simulink model "model"  (R2016a)
(part 2 of 2)

  bus74 : powerlib/Measurements/Load Flow Bus  LConnTagsString=a  Phases=single  Connectors=on one side  ID=bus74  Vbase=225000  Vref=1  Vangle=0  VLF=1  VLFb=1  VLFc=1  angleLF=0  angleLFb=0  angleLFc=0
      settings: AttributesFormatString=|
      | %<ID>
      | %<Vbase>V
      | %<VLF>pu
      | %<angleLF>deg.
      | %<Name>
  bus75 : powerlib/Measurements/Load Flow Bus  LConnTagsString=a  Phases=single  Connectors=on one side  ID=bus75  Vbase=225000  Vref=1  Vangle=0  VLF=1  VLFb=1  VLFc=1  angleLF=0  angleLFb=0  angleLFc=0
      settings: AttributesFormatString=|
      | %<ID>
      | %<Vbase>V
      | %<VLF>pu
      | %<angleLF>deg.
      | %<Name>
  bus76 : powerlib/Measurements/Load Flow Bus  LConnTagsString=a  Phases=single  Connectors=on one side  ID=bus76  Vbase=225000  Vref=1  Vangle=0  VLF=1  VLFb=1  VLFc=1  angleLF=0  angleLFb=0  angleLFc=0
      settings: AttributesFormatString=|
      | %<ID>
      | %<Vbase>V
      | %<VLF>pu
      | %<angleLF>deg.
      | %<Name>
  bus77 : powerlib/Measurements/Load Flow Bus  LConnTagsString=a  Phases=single  Connectors=on one side  ID=bus77  Vbase=225000  Vref=1  Vangle=0  VLF=1  VLFb=1  VLFc=1  angleLF=0  angleLFb=0  angleLFc=0
      settings: AttributesFormatString=|
      | %<ID>
      | %<Vbase>V
      | %<VLF>pu
      | %<angleLF>deg.
      | %<Name>
  bus78 : powerlib/Measurements/Load Flow Bus  LConnTagsString=a  Phases=single  Connectors=on one side  ID=bus78  Vbase=225000  Vref=1  Vangle=0  VLF=1  VLFb=1  VLFc=1  angleLF=0  angleLFb=0  angleLFc=0
      settings: AttributesFormatString=|
      | %<ID>
      | %<Vbase>V
      | %<VLF>pu
      | %<angleLF>deg.
      | %<Name>
  bus79 : powerlib/Measurements/Load Flow Bus  LConnTagsString=a  Phases=single  Connectors=on one side  ID=bus79  Vbase=225000  Vref=1  Vangle=0  VLF=1  VLFb=1  VLFc=1  angleLF=0  angleLFb=0  angleLFc=0
      settings: AttributesFormatString=|
      | %<ID>
      | %<Vbase>V
      | %<VLF>pu
      | %<angleLF>deg.
      | %<Name>
  bus8 : powerlib/Measurements/Load Flow Bus  LConnTagsString=a  Phases=single  Connectors=on one side  ID=bus8  Vbase=225000  Vref=1  Vangle=0  VLF=1  VLFb=1  VLFc=1  angleLF=0  angleLFb=0  angleLFc=0
      settings: AttributesFormatString=|
      | %<ID>
      | %<Vbase>V
      | %<VLF>pu
      | %<angleLF>deg.
      | %<Name>
  bus80 : powerlib/Measurements/Load Flow Bus  LConnTagsString=a  Phases=single  Connectors=on one side  ID=bus80  Vbase=225000  Vref=1  Vangle=0  VLF=1  VLFb=1  VLFc=1  angleLF=0  angleLFb=0  angleLFc=0
      settings: AttributesFormatString=|
      | %<ID>
      | %<Vbase>V
      | %<VLF>pu
      | %<angleLF>deg.
      | %<Name>
  bus81 : powerlib/Measurements/Load Flow Bus  LConnTagsString=a  Phases=single  Connectors=on one side  ID=bus81  Vbase=225000  Vref=1  Vangle=0  VLF=1  VLFb=1  VLFc=1  angleLF=0  angleLFb=0  angleLFc=0
      settings: AttributesFormatString=|
      | %<ID>
      | %<Vbase>V
      | %<VLF>pu
      | %<angleLF>deg.
      | %<Name>
  bus82 : powerlib/Measurements/Load Flow Bus  LConnTagsString=a  Phases=single  Connectors=on one side  ID=bus82  Vbase=225000  Vref=1  Vangle=0  VLF=1  VLFb=1  VLFc=1  angleLF=0  angleLFb=0  angleLFc=0
      settings: AttributesFormatString=|
      | %<ID>
      | %<Vbase>V
      | %<VLF>pu
      | %<angleLF>deg.
      | %<Name>
  bus83 : powerlib/Measurements/Load Flow Bus  LConnTagsString=a  Phases=single  Connectors=on one side  ID=bus83  Vbase=225000  Vref=1  Vangle=0  VLF=1  VLFb=1  VLFc=1  angleLF=0  angleLFb=0  angleLFc=0
      settings: AttributesFormatString=|
      | %<ID>
      | %<Vbase>V
      | %<VLF>pu
      | %<angleLF>deg.
      | %<Name>
  bus84 : powerlib/Measurements/Load Flow Bus  LConnTagsString=a  Phases=single  Connectors=on one side  ID=bus84  Vbase=225000  Vref=1  Vangle=0  VLF=1  VLFb=1  VLFc=1  angleLF=0  angleLFb=0  angleLFc=0
      settings: AttributesFormatString=|
      | %<ID>
      | %<Vbase>V
      | %<VLF>pu
      | %<angleLF>deg.
      | %<Name>
  bus85 : powerlib/Measurements/Load Flow Bus  LConnTagsString=a  Phases=single  Connectors=on one side  ID=bus85  Vbase=225000  Vref=1  Vangle=0  VLF=1  VLFb=1  VLFc=1  angleLF=0  angleLFb=0  angleLFc=0
      settings: AttributesFormatString=|
      | %<ID>
      | %<Vbase>V
      | %<VLF>pu
      | %<angleLF>deg.
      | %<Name>
  bus86 : powerlib/Measurements/Load Flow Bus  LConnTagsString=a  Phases=single  Connectors=on one side  ID=bus86  Vbase=225000  Vref=1  Vangle=0  VLF=1  VLFb=1  VLFc=1  angleLF=0  angleLFb=0  angleLFc=0
      settings: AttributesFormatString=|
      | %<ID>
      | %<Vbase>V
      | %<VLF>pu
      | %<angleLF>deg.
      | %<Name>
  bus87 : powerlib/Measurements/Load Flow Bus  LConnTagsString=a  Phases=single  Connectors=on one side  ID=bus87  Vbase=225000  Vref=1  Vangle=0  VLF=1  VLFb=1  VLFc=1  angleLF=0  angleLFb=0  angleLFc=0
      settings: AttributesFormatString=|
      | %<ID>
      | %<Vbase>V
      | %<VLF>pu
      | %<angleLF>deg.
      | %<Name>
  bus88 : powerlib/Measurements/Load Flow Bus  LConnTagsString=a  Phases=single  Connectors=on one side  ID=bus88  Vbase=225000  Vref=1  Vangle=0  VLF=1  VLFb=1  VLFc=1  angleLF=0  angleLFb=0  angleLFc=0
      settings: AttributesFormatString=|
      | %<ID>
      | %<Vbase>V
      | %<VLF>pu
      | %<angleLF>deg.
      | %<Name>
  bus89 : powerlib/Measurements/Load Flow Bus  LConnTagsString=a  Phases=single  Connectors=on one side  ID=bus89  Vbase=225000  Vref=1  Vangle=0  VLF=1  VLFb=1  VLFc=1  angleLF=0  angleLFb=0  angleLFc=0
      settings: AttributesFormatString=|
      | %<ID>
      | %<Vbase>V
      | %<VLF>pu
      | %<angleLF>deg.
      | %<Name>
  bus9 : powerlib/Measurements/Load Flow Bus  LConnTagsString=a  Phases=single  Connectors=on one side  ID=bus9  Vbase=225000  Vref=1  Vangle=0  VLF=1  VLFb=1  VLFc=1  angleLF=0  angleLFb=0  angleLFc=0
      settings: AttributesFormatString=|
      | %<ID>
      | %<Vbase>V
      | %<VLF>pu
      | %<angleLF>deg.
      | %<Name>
  bus90 : powerlib/Measurements/Load Flow Bus  LConnTagsString=a  Phases=single  Connectors=on one side  ID=bus90  Vbase=225000  Vref=1  Vangle=0  VLF=1  VLFb=1  VLFc=1  angleLF=0  angleLFb=0  angleLFc=0
      settings: AttributesFormatString=|
      | %<ID>
      | %<Vbase>V
      | %<VLF>pu
      | %<angleLF>deg.
      | %<Name>
  bus91 : powerlib/Measurements/Load Flow Bus  LConnTagsString=a  Phases=single  Connectors=on one side  ID=bus91  Vbase=225000  Vref=1  Vangle=0  VLF=1  VLFb=1  VLFc=1  angleLF=0  angleLFb=0  angleLFc=0
      settings: AttributesFormatString=|
      | %<ID>
      | %<Vbase>V
      | %<VLF>pu
      | %<angleLF>deg.
      | %<Name>
  bus92 : powerlib/Measurements/Load Flow Bus  LConnTagsString=a  Phases=single  Connectors=on one side  ID=bus92  Vbase=225000  Vref=1  Vangle=0  VLF=1  VLFb=1  VLFc=1  angleLF=0  angleLFb=0  angleLFc=0
      settings: AttributesFormatString=|
      | %<ID>
      | %<Vbase>V
      | %<VLF>pu
      | %<angleLF>deg.
      | %<Name>
  bus93 : powerlib/Measurements/Load Flow Bus  LConnTagsString=a  Phases=single  Connectors=on one side  ID=bus93  Vbase=225000  Vref=1  Vangle=0  VLF=1  VLFb=1  VLFc=1  angleLF=0  angleLFb=0  angleLFc=0
      settings: AttributesFormatString=|
      | %<ID>
      | %<Vbase>V
      | %<VLF>pu
      | %<angleLF>deg.
      | %<Name>
  bus94 : powerlib/Measurements/Load Flow Bus  LConnTagsString=a  Phases=single  Connectors=on one side  ID=bus94  Vbase=225000  Vref=1  Vangle=0  VLF=1  VLFb=1  VLFc=1  angleLF=0  angleLFb=0  angleLFc=0
      settings: AttributesFormatString=|
      | %<ID>
      | %<Vbase>V
      | %<VLF>pu
      | %<angleLF>deg.
      | %<Name>
  bus95 : powerlib/Measurements/Load Flow Bus  LConnTagsString=a  Phases=single  Connectors=on one side  ID=bus95  Vbase=225000  Vref=1  Vangle=0  VLF=1  VLFb=1  VLFc=1  angleLF=0  angleLFb=0  angleLFc=0
      settings: AttributesFormatString=|
      | %<ID>
      | %<Vbase>V
      | %<VLF>pu
      | %<angleLF>deg.
      | %<Name>
  bus96 : powerlib/Measurements/Load Flow Bus  LConnTagsString=a  Phases=single  Connectors=on one side  ID=bus96  Vbase=225000  Vref=1  Vangle=0  VLF=1  VLFb=1  VLFc=1  angleLF=0  angleLFb=0  angleLFc=0
      settings: AttributesFormatString=|
      | %<ID>
      | %<Vbase>V
      | %<VLF>pu
      | %<angleLF>deg.
      | %<Name>
  bus97 : powerlib/Measurements/Load Flow Bus  LConnTagsString=a  Phases=single  Connectors=on one side  ID=bus97  Vbase=225000  Vref=1  Vangle=0  VLF=1  VLFb=1  VLFc=1  angleLF=0  angleLFb=0  angleLFc=0
      settings: AttributesFormatString=|
      | %<ID>
      | %<Vbase>V
      | %<VLF>pu
      | %<angleLF>deg.
      | %<Name>
  bus98 : powerlib/Measurements/Load Flow Bus  LConnTagsString=a  Phases=single  Connectors=on one side  ID=bus98  Vbase=225000  Vref=1  Vangle=0  VLF=1  VLFb=1  VLFc=1  angleLF=0  angleLFb=0  angleLFc=0
      settings: AttributesFormatString=|
      | %<ID>
      | %<Vbase>V
      | %<VLF>pu
      | %<angleLF>deg.
      | %<Name>
  bus99 : powerlib/Measurements/Load Flow Bus  LConnTagsString=a  Phases=single  Connectors=on one side  ID=bus99  Vbase=225000  Vref=1  Vangle=0  VLF=1  VLFb=1  VLFc=1  angleLF=0  angleLFb=0  angleLFc=0
      settings: AttributesFormatString=|
      | %<ID>
      | %<Vbase>V
      | %<VLF>pu
      | %<angleLF>deg.
      | %<Name>
  powergui : powerlib/powergui  Priority=1  SimulationMode=Phasor  SolverType=Tustin/Backward Euler (TBE)  SampleTime=50e-6  frequency=50  SPID=off  DisableSnubberDevices=off  DisableRonSwitches=off  DisableVfSwitches=off  SwTol=0  DisplayEquations=off  Interpol=off  ExternalGateDelay=off  methode=off  Ts=10  FunctionMessages=off  echomessages=off  HookPort=off  EnableUseOfTLC=off  x0status=blocks  frequencyindice=50  Pbase=3000e6  ErrMax=0.0001  Iterations=50  UnitsV=V  UnitsW=W  buscounter=0  RestoreLinks=warning  ResistiveCurrentMeasurement=off  Frange=[0:2:500]  Ylog=off  Xlog=on  ShowGrid=off  save=off  variable=ZData  structure=0  ZoomFFT=off  StartTime=0.0  cycles=1  DisplayStyle=1  fundamental=60  FreqAxis=off  MaxFrequency=1000  frequencyindicesteady=1  RmsSteady=1  display=off
  connections:
  _CN_200906153_225000_CN_250878457_225000/LConn1 -- T_200906153_225000_/LConn1 -- _CN_200906153_225000_CN_285708473_225000/LConn1 -- _CN_200906153_225000_CN_218739270_225000/LConn1 -- _CN_200906153_225000_CN_271316486_225000/LConn1
  _CN_200906153_225000_CN_250878457_225000/LConn2 -- T_200906153_225000_/LConn2 -- _CN_200906153_225000_CN_285708473_225000/LConn2 -- _CN_200906153_225000_CN_218739270_225000/LConn2 -- _CN_200906153_225000_CN_271316486_225000/LConn2
  _CN_200906153_225000_CN_250878457_225000/LConn3 -- T_200906153_225000_/LConn3 -- _CN_200906153_225000_CN_285708473_225000/LConn3 -- _CN_200906153_225000_CN_218739270_225000/LConn3 -- _CN_200906153_225000_CN_271316486_225000/LConn3 -- bus1/LConn1
  _CN_200906153_225000_CN_250878457_225000/RConn1 -- T_250878457_225000_/LConn1 -- _CN_94548360_225000_CN_250878457_225000/LConn1 -- _CN_208002693_225000_CN_250878457_225000/LConn1
  _CN_200906153_225000_CN_250878457_225000/RConn2 -- T_250878457_225000_/LConn2 -- _CN_94548360_225000_CN_250878457_225000/LConn2 -- _CN_208002693_225000_CN_250878457_225000/LConn2
  _CN_200906153_225000_CN_250878457_225000/RConn3 -- T_250878457_225000_/LConn3 -- _CN_94548360_225000_CN_250878457_225000/LConn3 -- bus2/LConn1 -- _CN_208002693_225000_CN_250878457_225000/LConn3
  T_285708473_225000_/LConn1 -- _CN_200906153_225000_CN_285708473_225000/RConn1
  T_285708473_225000_/LConn2 -- _CN_200906153_225000_CN_285708473_225000/RConn2
  _CN_200906153_225000_CN_285708473_225000/RConn3 -- T_285708473_225000_/LConn3 -- bus3/LConn1
  T_218739270_225000_/LConn1 -- _CN_200906153_225000_CN_218739270_225000/RConn1
  T_218739270_225000_/LConn2 -- _CN_200906153_225000_CN_218739270_225000/RConn2
  _CN_200906153_225000_CN_218739270_225000/RConn3 -- T_218739270_225000_/LConn3 -- bus4/LConn1
  T_271316486_225000_/LConn1 -- _CN_200906153_225000_CN_271316486_225000/RConn1
  T_271316486_225000_/LConn2 -- _CN_200906153_225000_CN_271316486_225000/RConn2
  _CN_200906153_225000_CN_271316486_225000/RConn3 -- T_271316486_225000_/LConn3 -- bus5/LConn1
  _CN_97706499_225000_CN_215403934_225000/LConn1 -- T_97706499_225000_/RConn1 -- _CN_97706499_225000_CN_94548360_225000/LConn1 -- L_97706499/LConn1 -- _CN_97706499_225000_CN_320483882_225000/LConn1 -- _CN_97706499_225000_CN_316738277_225000/LConn1 -- _CN_97706499_225000_CN_200913450_225000/LConn1 -- _CN_97706499_225000_CN_182345278_225000/LConn1
  _CN_97706499_225000_CN_215403934_225000/LConn2 -- T_97706499_225000_/RConn2 -- _CN_97706499_225000_CN_94548360_225000/LConn2 -- L_97706499/LConn2 -- _CN_97706499_225000_CN_320483882_225000/LConn2 -- _CN_97706499_225000_CN_316738277_225000/LConn2 -- _CN_97706499_225000_CN_200913450_225000/LConn2 -- _CN_97706499_225000_CN_182345278_225000/LConn2
  _CN_97706499_225000_CN_215403934_225000/LConn3 -- T_97706499_225000_/RConn3 -- _CN_97706499_225000_CN_94548360_225000/LConn3 -- L_97706499/LConn3 -- bus6/LConn1 -- _CN_97706499_225000_CN_320483882_225000/LConn3 -- _CN_97706499_225000_CN_316738277_225000/LConn3 -- _CN_97706499_225000_CN_200913450_225000/LConn3 -- _CN_97706499_225000_CN_182345278_225000/LConn3
  _CN_97706499_225000_CN_215403934_225000/RConn1 -- T_215403934_225000_/LConn1 -- _CN_94548360_225000_CN_215403934_225000/LConn1
  _CN_97706499_225000_CN_215403934_225000/RConn2 -- T_215403934_225000_/LConn2 -- _CN_94548360_225000_CN_215403934_225000/LConn2
  _CN_97706499_225000_CN_215403934_225000/RConn3 -- T_215403934_225000_/LConn3 -- _CN_94548360_225000_CN_215403934_225000/LConn3 -- bus7/LConn1
  T_320483882_225000_/LConn1 -- _CN_97706499_225000_CN_320483882_225000/RConn1
  T_320483882_225000_/LConn2 -- _CN_97706499_225000_CN_320483882_225000/RConn2
  _CN_97706499_225000_CN_320483882_225000/RConn3 -- T_320483882_225000_/LConn3 -- bus8/LConn1
  _CN_97706499_225000_CN_316738277_225000/RConn1 -- T_316738277__/RConn1 -- L_316738277/LConn1
  _CN_97706499_225000_CN_316738277_225000/RConn2 -- T_316738277__/RConn2 -- L_316738277/LConn2
  _CN_97706499_225000_CN_316738277_225000/RConn3 -- T_316738277__/RConn3 -- L_316738277/LConn3 -- bus9/LConn1
  _CN_97706499_225000_CN_200913450_225000/RConn1 -- T_200913450_225000_/LConn1 -- _CN_200913450_225000_CN_200915133_225000/LConn1 -- _CN_200913450_225000_CN_197830862_225000/LConn1
  _CN_97706499_225000_CN_200913450_225000/RConn2 -- T_200913450_225000_/LConn2 -- _CN_200913450_225000_CN_200915133_225000/LConn2 -- _CN_200913450_225000_CN_197830862_225000/LConn2
  _CN_97706499_225000_CN_200913450_225000/RConn3 -- T_200913450_225000_/LConn3 -- _CN_200913450_225000_CN_200915133_225000/LConn3 -- _CN_200913450_225000_CN_197830862_225000/LConn3 -- bus10/LConn1
  _CN_97706499_225000_CN_182345278_225000/RConn1 -- T_182345278_225000_/LConn1 -- _CN_200915133_225000_CN_182345278_225000/LConn1
  _CN_97706499_225000_CN_182345278_225000/RConn2 -- T_182345278_225000_/LConn2 -- _CN_200915133_225000_CN_182345278_225000/LConn2
  _CN_97706499_225000_CN_182345278_225000/RConn3 -- T_182345278_225000_/LConn3 -- _CN_200915133_225000_CN_182345278_225000/LConn3 -- bus11/LConn1
  _CN_97706499_225000_CN_94548360_225000/RConn1 -- T_94548360_225000_/LConn1 -- _CN_94548360_225000_CN_215403934_225000/RConn1 -- _CN_94548360_225000_CN_250878457_225000/RConn1
  _CN_97706499_225000_CN_94548360_225000/RConn2 -- T_94548360_225000_/LConn2 -- _CN_94548360_225000_CN_215403934_225000/RConn2 -- _CN_94548360_225000_CN_250878457_225000/RConn2
  _CN_97706499_225000_CN_94548360_225000/RConn3 -- T_94548360_225000_/LConn3 -- _CN_94548360_225000_CN_215403934_225000/RConn3 -- bus12/LConn1 -- _CN_94548360_225000_CN_250878457_225000/RConn3
  _CN_208002693_225000_CN_108482559_225000/LConn1 -- T_208002693_225000_/LConn1 -- _CN_208002693_225000_CN_250878457_225000/RConn1 -- _CN_208002693_225000_CN_131995387_225000/LConn1
  _CN_208002693_225000_CN_108482559_225000/LConn2 -- T_208002693_225000_/LConn2 -- _CN_208002693_225000_CN_250878457_225000/RConn2 -- _CN_208002693_225000_CN_131995387_225000/LConn2
  _CN_208002693_225000_CN_108482559_225000/LConn3 -- T_208002693_225000_/LConn3 -- _CN_208002693_225000_CN_250878457_225000/RConn3 -- _CN_208002693_225000_CN_131995387_225000/LConn3 -- bus13/LConn1
  T_108482559_225000_/LConn1 -- _CN_208002693_225000_CN_108482559_225000/RConn1
  T_108482559_225000_/LConn2 -- _CN_208002693_225000_CN_108482559_225000/RConn2
  _CN_208002693_225000_CN_108482559_225000/RConn3 -- T_108482559_225000_/LConn3 -- bus14/LConn1
  _CN_208002693_225000_CN_131995387_225000/RConn1 -- T_131995387_225000_/LConn1 -- _CN_131992905_225000_CN_131995387_225000/LConn1 -- _CN_131995387_225000_CN_131408509_225000/LConn1
  _CN_208002693_225000_CN_131995387_225000/RConn2 -- T_131995387_225000_/LConn2 -- _CN_131992905_225000_CN_131995387_225000/LConn2 -- _CN_131995387_225000_CN_131408509_225000/LConn2
  _CN_208002693_225000_CN_131995387_225000/RConn3 -- T_131995387_225000_/LConn3 -- _CN_131992905_225000_CN_131995387_225000/LConn3 -- _CN_131995387_225000_CN_131408509_225000/LConn3 -- bus15/LConn1
  _CN_131891079_225000_CN_131892127_225000/LConn1 -- T_131891079_225000;60000_/LConn1 -- _CN_131891079_225000_CN_95436126_225000/LConn1 -- _CN_131891079_225000_CN_207991977_225000/LConn1 -- _CN_131891079_225000_CN_131946012_225000/LConn1 -- _CN_131891079_225000_CN_131408509_225000/LConn1 -- _CN_131891079_225000_CN_131588990_225000/LConn1 -- _CN_131891079_225000_CN_131267165_225000/LConn1 -- _CN_131891079_225000_CN_143628748_225000/LConn1 -- _CN_131891079_225000_CN_131902940_225000/LConn1
  _CN_131891079_225000_CN_131892127_225000/LConn2 -- T_131891079_225000;60000_/LConn2 -- _CN_131891079_225000_CN_95436126_225000/LConn2 -- _CN_131891079_225000_CN_207991977_225000/LConn2 -- _CN_131891079_225000_CN_131946012_225000/LConn2 -- _CN_131891079_225000_CN_131408509_225000/LConn2 -- _CN_131891079_225000_CN_131588990_225000/LConn2 -- _CN_131891079_225000_CN_131267165_225000/LConn2 -- _CN_131891079_225000_CN_143628748_225000/LConn2 -- _CN_131891079_225000_CN_131902940_225000/LConn2
  _CN_131891079_225000_CN_131892127_225000/LConn3 -- T_131891079_225000;60000_/LConn3 -- _CN_131891079_225000_CN_95436126_225000/LConn3 -- bus16/LConn1 -- _CN_131891079_225000_CN_207991977_225000/LConn3 -- _CN_131891079_225000_CN_131946012_225000/LConn3 -- _CN_131891079_225000_CN_131408509_225000/LConn3 -- _CN_131891079_225000_CN_131588990_225000/LConn3 -- _CN_131891079_225000_CN_131267165_225000/LConn3 -- _CN_131891079_225000_CN_143628748_225000/LConn3 -- _CN_131891079_225000_CN_131902940_225000/LConn3
  _CN_131891079_225000_CN_131892127_225000/RConn1 -- T_131892127_225000;60000_/LConn1 -- _CN_131892127_225000_CN_95436126_225000/LConn1 -- _CN_131892127_225000_CN_131893727_225000/LConn1 -- _CN_131892127_225000_CN_131899192_225000/LConn1
  _CN_131891079_225000_CN_131892127_225000/RConn2 -- T_131892127_225000;60000_/LConn2 -- _CN_131892127_225000_CN_95436126_225000/LConn2 -- _CN_131892127_225000_CN_131893727_225000/LConn2 -- _CN_131892127_225000_CN_131899192_225000/LConn2
  _CN_131891079_225000_CN_131892127_225000/RConn3 -- T_131892127_225000;60000_/LConn3 -- _CN_131892127_225000_CN_95436126_225000/LConn3 -- _CN_131892127_225000_CN_131893727_225000/LConn3 -- bus17/LConn1 -- _CN_131892127_225000_CN_131899192_225000/LConn3
  _CN_131891079_225000_CN_207991977_225000/RConn1 -- T_207991977_225000_/LConn1 -- _CN_131899192_225000_CN_207991977_225000/LConn1
  _CN_131891079_225000_CN_207991977_225000/RConn2 -- T_207991977_225000_/LConn2 -- _CN_131899192_225000_CN_207991977_225000/LConn2
  _CN_131891079_225000_CN_207991977_225000/RConn3 -- T_207991977_225000_/LConn3 -- _CN_131899192_225000_CN_207991977_225000/LConn3 -- bus18/LConn1
  _CN_131891079_225000_CN_131946012_225000/RConn1 -- T_131946012_400000;225000_/RConn1 -- _CN_131946012_225000_CN_144011573_225000/LConn1 -- _CN_131946012_225000_CN_207995370_225000/LConn1 -- _CN_131946012_225000_CN_207997682_225000/LConn1 -- _CN_131946012_225000_CN_131902940_225000/LConn1 -- L_131946012/LConn1
  _CN_131891079_225000_CN_131946012_225000/RConn2 -- T_131946012_400000;225000_/RConn2 -- _CN_131946012_225000_CN_144011573_225000/LConn2 -- _CN_131946012_225000_CN_207995370_225000/LConn2 -- _CN_131946012_225000_CN_207997682_225000/LConn2 -- _CN_131946012_225000_CN_131902940_225000/LConn2 -- L_131946012/LConn2
  _CN_131891079_225000_CN_131946012_225000/RConn3 -- T_131946012_400000;225000_/RConn3 -- _CN_131946012_225000_CN_144011573_225000/LConn3 -- _CN_131946012_225000_CN_207995370_225000/LConn3 -- _CN_131946012_225000_CN_207997682_225000/LConn3 -- _CN_131946012_225000_CN_131902940_225000/LConn3 -- L_131946012/LConn3 -- bus19/LConn1
  _CN_131891079_225000_CN_131408509_225000/RConn1 -- T_131408509_225000_/LConn1 -- _CN_142520745_225000_CN_131408509_225000/LConn1 -- _CN_131995387_225000_CN_131408509_225000/RConn1 -- _CN_131408509_225000_CN_131267165_225000/LConn1
  _CN_131891079_225000_CN_131408509_225000/RConn2 -- T_131408509_225000_/LConn2 -- _CN_142520745_225000_CN_131408509_225000/LConn2 -- _CN_131995387_225000_CN_131408509_225000/RConn2 -- _CN_131408509_225000_CN_131267165_225000/LConn2
  _CN_131891079_225000_CN_131408509_225000/RConn3 -- T_131408509_225000_/LConn3 -- _CN_142520745_225000_CN_131408509_225000/LConn3 -- _CN_131995387_225000_CN_131408509_225000/RConn3 -- _CN_131408509_225000_CN_131267165_225000/LConn3 -- bus20/LConn1
  _CN_131891079_225000_CN_131588990_225000/RConn1 -- T_131588990_225000;60000_/LConn1 -- _CN_131591106_225000_CN_131588990_225000/LConn1
  _CN_131891079_225000_CN_131588990_225000/RConn2 -- T_131588990_225000;60000_/LConn2 -- _CN_131591106_225000_CN_131588990_225000/LConn2
  _CN_131891079_225000_CN_131588990_225000/RConn3 -- T_131588990_225000;60000_/LConn3 -- _CN_131591106_225000_CN_131588990_225000/LConn3 -- bus21/LConn1
  _CN_131891079_225000_CN_131267165_225000/RConn1 -- G_131267165_/RConn1 -- _CN_131408509_225000_CN_131267165_225000/RConn1
  _CN_131891079_225000_CN_131267165_225000/RConn2 -- G_131267165_/RConn2 -- _CN_131408509_225000_CN_131267165_225000/RConn2
  _CN_131891079_225000_CN_131267165_225000/RConn3 -- G_131267165_/RConn3 -- _CN_131408509_225000_CN_131267165_225000/RConn3 -- bus22/LConn1
  _CN_131891079_225000_CN_143628748_225000/RConn1 -- T_143628748_225000_/LConn1 -- _CN_131591106_225000_CN_143628748_225000/LConn1
  _CN_131891079_225000_CN_143628748_225000/RConn2 -- T_143628748_225000_/LConn2 -- _CN_131591106_225000_CN_143628748_225000/LConn2
  _CN_131891079_225000_CN_143628748_225000/RConn3 -- T_143628748_225000_/LConn3 -- _CN_131591106_225000_CN_143628748_225000/LConn3 -- bus23/LConn1
  _CN_131891079_225000_CN_131902940_225000/RConn1 -- T_131902940_225000_/LConn1 -- _CN_131946012_225000_CN_131902940_225000/RConn1 -- _CN_131902940_225000_CN_131947753_225000/LConn1
  _CN_131891079_225000_CN_131902940_225000/RConn2 -- T_131902940_225000_/LConn2 -- _CN_131946012_225000_CN_131902940_225000/RConn2 -- _CN_131902940_225000_CN_131947753_225000/LConn2
  _CN_131891079_225000_CN_131902940_225000/RConn3 -- T_131902940_225000_/LConn3 -- _CN_131946012_225000_CN_131902940_225000/RConn3 -- _CN_131902940_225000_CN_131947753_225000/LConn3 -- bus24/LConn1
  _CN_131891079_225000_CN_95436126_225000/RConn1 -- T_95436126_225000;60000_/LConn1 -- _CN_143685412_225000_CN_95436126_225000/LConn1 -- _CN_167920552_225000_CN_95436126_225000/LConn1 -- _CN_143699506_225000_CN_95436126_225000/LConn1 -- _CN_95436126_225000_CN_251222750_225000/LConn1 -- _CN_95436126_225000_CN_143752299_225000/LConn1 -- _CN_131892127_225000_CN_95436126_225000/RConn1 -- _CN_163471767_225000_CN_95436126_225000/LConn1
  _CN_131891079_225000_CN_95436126_225000/RConn2 -- T_95436126_225000;60000_/LConn2 -- _CN_143685412_225000_CN_95436126_225000/LConn2 -- _CN_167920552_225000_CN_95436126_225000/LConn2 -- _CN_143699506_225000_CN_95436126_225000/LConn2 -- _CN_95436126_225000_CN_251222750_225000/LConn2 -- _CN_95436126_225000_CN_143752299_225000/LConn2 -- _CN_131892127_225000_CN_95436126_225000/RConn2 -- _CN_163471767_225000_CN_95436126_225000/LConn2
  _CN_131891079_225000_CN_95436126_225000/RConn3 -- T_95436126_225000;60000_/LConn3 -- _CN_143685412_225000_CN_95436126_225000/LConn3 -- _CN_167920552_225000_CN_95436126_225000/LConn3 -- _CN_143699506_225000_CN_95436126_225000/LConn3 -- _CN_95436126_225000_CN_251222750_225000/LConn3 -- _CN_95436126_225000_CN_143752299_225000/LConn3 -- bus25/LConn1 -- _CN_131892127_225000_CN_95436126_225000/RConn3 -- _CN_163471767_225000_CN_95436126_225000/LConn3
  _CN_163471767_225000_CN_95436126_225000/RConn1 -- T_163471767_225000_/LConn1 -- _CN_163471767_225000_CN_163508115_225000/LConn1
  _CN_163471767_225000_CN_95436126_225000/RConn2 -- T_163471767_225000_/LConn2 -- _CN_163471767_225000_CN_163508115_225000/LConn2
  _CN_163471767_225000_CN_95436126_225000/RConn3 -- T_163471767_225000_/LConn3 -- _CN_163471767_225000_CN_163508115_225000/LConn3 -- bus26/LConn1
  _CN_163471767_225000_CN_163508115_225000/RConn1 -- G_163508115_Allal_al_Fassi_Hydroelectric_Plant/RConn1 -- _CN_143685412_225000_CN_163508115_225000/LConn1
  _CN_163471767_225000_CN_163508115_225000/RConn2 -- G_163508115_Allal_al_Fassi_Hydroelectric_Plant/RConn2 -- _CN_143685412_225000_CN_163508115_225000/LConn2
  _CN_163471767_225000_CN_163508115_225000/RConn3 -- G_163508115_Allal_al_Fassi_Hydroelectric_Plant/RConn3 -- _CN_143685412_225000_CN_163508115_225000/LConn3 -- bus27/LConn1
  _CN_143736898_225000_CN_143752299_225000/LConn1 -- T_143736898__/LConn1 -- _CN_143736898_225000_CN_167406532_225000/LConn1
  _CN_143736898_225000_CN_143752299_225000/LConn2 -- T_143736898__/LConn2 -- _CN_143736898_225000_CN_167406532_225000/LConn2
  _CN_143736898_225000_CN_143752299_225000/LConn3 -- T_143736898__/LConn3 -- _CN_143736898_225000_CN_167406532_225000/LConn3 -- bus28/LConn1
  _CN_143736898_225000_CN_143752299_225000/RConn1 -- T_143752299_400000;225000_/LConn1 -- _CN_167406532_225000_CN_143752299_225000/LConn1 -- _CN_95436126_225000_CN_143752299_225000/RConn1 -- _CN_143752299_225000_CN_150122664_225000/LConn1 -- _CN_208137370_225000_CN_143752299_225000/LConn1
  _CN_143736898_225000_CN_143752299_225000/RConn2 -- T_143752299_400000;225000_/LConn2 -- _CN_167406532_225000_CN_143752299_225000/LConn2 -- _CN_95436126_225000_CN_143752299_225000/RConn2 -- _CN_143752299_225000_CN_150122664_225000/LConn2 -- _CN_208137370_225000_CN_143752299_225000/LConn2
  _CN_143736898_225000_CN_143752299_225000/RConn3 -- T_143752299_400000;225000_/LConn3 -- _CN_167406532_225000_CN_143752299_225000/LConn3 -- _CN_95436126_225000_CN_143752299_225000/RConn3 -- _CN_143752299_225000_CN_150122664_225000/LConn3 -- bus29/LConn1 -- _CN_208137370_225000_CN_143752299_225000/LConn3
  _CN_143736898_225000_CN_167406532_225000/RConn1 -- T_167406532_225000_/LConn1 -- _CN_167406532_225000_CN_143752299_225000/RConn1 -- _CN_167406532_225000_CN_207823867_225000/LConn1
  _CN_143736898_225000_CN_167406532_225000/RConn2 -- T_167406532_225000_/LConn2 -- _CN_167406532_225000_CN_143752299_225000/RConn2 -- _CN_167406532_225000_CN_207823867_225000/LConn2
  _CN_143736898_225000_CN_167406532_225000/RConn3 -- T_167406532_225000_/LConn3 -- _CN_167406532_225000_CN_143752299_225000/RConn3 -- _CN_167406532_225000_CN_207823867_225000/LConn3 -- bus30/LConn1
  _CN_143681023_225000_CN_96831672_225000/LConn1 -- T_143681023_225000;60000_/LConn1 -- _CN_143681023_225000_CN_359251299_225000/LConn1
  _CN_143681023_225000_CN_96831672_225000/LConn2 -- T_143681023_225000;60000_/LConn2 -- _CN_143681023_225000_CN_359251299_225000/LConn2
  _CN_143681023_225000_CN_96831672_225000/LConn3 -- T_143681023_225000;60000_/LConn3 -- _CN_143681023_225000_CN_359251299_225000/LConn3 -- bus31/LConn1
  _CN_143681023_225000_CN_96831672_225000/RConn1 -- T_96831672_225000_/LConn1 -- _CN_144011974_225000_CN_96831672_225000/LConn1
  _CN_143681023_225000_CN_96831672_225000/RConn2 -- T_96831672_225000_/LConn2 -- _CN_144011974_225000_CN_96831672_225000/LConn2
  _CN_143681023_225000_CN_96831672_225000/RConn3 -- T_96831672_225000_/LConn3 -- _CN_144011974_225000_CN_96831672_225000/LConn3 -- bus32/LConn1
  T_359251299__/LConn1 -- _CN_143681023_225000_CN_359251299_225000/RConn1
  T_359251299__/LConn2 -- _CN_143681023_225000_CN_359251299_225000/RConn2
  _CN_143681023_225000_CN_359251299_225000/RConn3 -- T_359251299__/LConn3 -- bus33/LConn1
  T_208137370_225000_/LConn1 -- _CN_208137370_225000_CN_143752299_225000/RConn1
  T_208137370_225000_/LConn2 -- _CN_208137370_225000_CN_143752299_225000/RConn2
  _CN_208137370_225000_CN_143752299_225000/RConn3 -- T_208137370_225000_/LConn3 -- bus34/LConn1
  _CN_131946012_225000_CN_144011573_225000/RConn1 -- T_144011573_225000;60000_/LConn1 -- _CN_144011573_225000_CN_131899192_225000/LConn1
  _CN_131946012_225000_CN_144011573_225000/RConn2 -- T_144011573_225000;60000_/LConn2 -- _CN_144011573_225000_CN_131899192_225000/LConn2
  _CN_131946012_225000_CN_144011573_225000/RConn3 -- T_144011573_225000;60000_/LConn3 -- _CN_144011573_225000_CN_131899192_225000/LConn3 -- bus35/LConn1
  T_207995370__/LConn1 -- _CN_131946012_225000_CN_207995370_225000/RConn1
  T_207995370__/LConn2 -- _CN_131946012_225000_CN_207995370_225000/RConn2
  _CN_131946012_225000_CN_207995370_225000/RConn3 -- T_207995370__/LConn3 -- bus36/LConn1
  _CN_131946012_225000_CN_207997682_225000/RConn1 -- T_207997682_225000;150000_/LConn1 -- _CN_216888494_225000_CN_207997682_225000/LConn1 -- _CN_131992905_225000_CN_207997682_225000/LConn1
  _CN_131946012_225000_CN_207997682_225000/RConn2 -- T_207997682_225000;150000_/LConn2 -- _CN_216888494_225000_CN_207997682_225000/LConn2 -- _CN_131992905_225000_CN_207997682_225000/LConn2
  _CN_131946012_225000_CN_207997682_225000/RConn3 -- T_207997682_225000;150000_/LConn3 -- _CN_216888494_225000_CN_207997682_225000/LConn3 -- _CN_131992905_225000_CN_207997682_225000/LConn3 -- bus37/LConn1
  _CN_131892127_225000_CN_131899192_225000/RConn1 -- T_131899192__/LConn1 -- _CN_144011573_225000_CN_131899192_225000/RConn1 -- _CN_131899192_225000_CN_207991977_225000/RConn1
  _CN_131892127_225000_CN_131899192_225000/RConn2 -- T_131899192__/LConn2 -- _CN_144011573_225000_CN_131899192_225000/RConn2 -- _CN_131899192_225000_CN_207991977_225000/RConn2
  _CN_131892127_225000_CN_131899192_225000/RConn3 -- T_131899192__/LConn3 -- _CN_144011573_225000_CN_131899192_225000/RConn3 -- _CN_131899192_225000_CN_207991977_225000/RConn3 -- bus38/LConn1
  T_131893727__/LConn1 -- _CN_131892127_225000_CN_131893727_225000/RConn1
  T_131893727__/LConn2 -- _CN_131892127_225000_CN_131893727_225000/RConn2
  _CN_131892127_225000_CN_131893727_225000/RConn3 -- T_131893727__/LConn3 -- bus39/LConn1
  _CN_143685412_225000_CN_163508115_225000/RConn1 -- T_143685412_225000_/LConn1 -- _CN_143685412_225000_CN_167920552_225000/LConn1 -- _CN_143685412_225000_CN_95436126_225000/RConn1
  _CN_143685412_225000_CN_163508115_225000/RConn2 -- T_143685412_225000_/LConn2 -- _CN_143685412_225000_CN_167920552_225000/LConn2 -- _CN_143685412_225000_CN_95436126_225000/RConn2
  _CN_143685412_225000_CN_163508115_225000/RConn3 -- T_143685412_225000_/LConn3 -- _CN_143685412_225000_CN_167920552_225000/LConn3 -- _CN_143685412_225000_CN_95436126_225000/RConn3 -- bus40/LConn1
  _CN_143685412_225000_CN_167920552_225000/RConn1 -- T_167920552_400000;225000_/RConn1 -- _CN_167920552_225000_CN_95436126_225000/RConn1 -- L_167920552/LConn1
  _CN_143685412_225000_CN_167920552_225000/RConn2 -- T_167920552_400000;225000_/RConn2 -- _CN_167920552_225000_CN_95436126_225000/RConn2 -- L_167920552/LConn2
  _CN_143685412_225000_CN_167920552_225000/RConn3 -- T_167920552_400000;225000_/RConn3 -- _CN_167920552_225000_CN_95436126_225000/RConn3 -- L_167920552/LConn3 -- bus41/LConn1
  T_142520745__/LConn1 -- _CN_142520745_225000_CN_131408509_225000/RConn1
  T_142520745__/LConn2 -- _CN_142520745_225000_CN_131408509_225000/RConn2
  _CN_142520745_225000_CN_131408509_225000/RConn3 -- T_142520745__/LConn3 -- bus42/LConn1
  _CN_200913450_225000_CN_200915133_225000/RConn1 -- T_200915133_225000_/LConn1 -- _CN_200915133_225000_CN_182345278_225000/RConn1
  _CN_200913450_225000_CN_200915133_225000/RConn2 -- T_200915133_225000_/LConn2 -- _CN_200915133_225000_CN_182345278_225000/RConn2
  _CN_200913450_225000_CN_200915133_225000/RConn3 -- T_200915133_225000_/LConn3 -- _CN_200915133_225000_CN_182345278_225000/RConn3 -- bus43/LConn1
  _CN_200913450_225000_CN_197830862_225000/RConn1 -- T_197830862__/LConn1 -- _CN_144011974_225000_CN_197830862_225000/LConn1
  _CN_200913450_225000_CN_197830862_225000/RConn2 -- T_197830862__/LConn2 -- _CN_144011974_225000_CN_197830862_225000/LConn2
  _CN_200913450_225000_CN_197830862_225000/RConn3 -- T_197830862__/LConn3 -- _CN_144011974_225000_CN_197830862_225000/LConn3 -- bus44/LConn1
  _CN_271334706_225000_CN_143699506_225000/LConn1 -- T_271334706__/LConn1 -- _CN_271334706_225000_CN_93147473_225000/LConn1
  _CN_271334706_225000_CN_143699506_225000/LConn2 -- T_271334706__/LConn2 -- _CN_271334706_225000_CN_93147473_225000/LConn2
  _CN_271334706_225000_CN_143699506_225000/LConn3 -- T_271334706__/LConn3 -- _CN_271334706_225000_CN_93147473_225000/LConn3 -- bus45/LConn1
  _CN_271334706_225000_CN_143699506_225000/RConn1 -- T_143699506_225000_/LConn1 -- _CN_143699506_225000_CN_166090341_225000/LConn1 -- _CN_143699506_225000_CN_95436126_225000/RConn1
  _CN_271334706_225000_CN_143699506_225000/RConn2 -- T_143699506_225000_/LConn2 -- _CN_143699506_225000_CN_166090341_225000/LConn2 -- _CN_143699506_225000_CN_95436126_225000/RConn2
  _CN_271334706_225000_CN_143699506_225000/RConn3 -- T_143699506_225000_/LConn3 -- _CN_143699506_225000_CN_166090341_225000/LConn3 -- bus46/LConn1 -- _CN_143699506_225000_CN_95436126_225000/RConn3
  _CN_271334706_225000_CN_93147473_225000/RConn1 -- T_93147473_400000;225000_/RConn1 -- _CN_93147473_225000_CN_131321800_225000/LConn1 -- _CN_93147473_225000_CN_131545712_225000/LConn1 -- L_93147473/LConn1 -- _CN_93147473_225000_CN_167908818_225000/LConn1
  _CN_271334706_225000_CN_93147473_225000/RConn2 -- T_93147473_400000;225000_/RConn2 -- _CN_93147473_225000_CN_131321800_225000/LConn2 -- _CN_93147473_225000_CN_131545712_225000/LConn2 -- L_93147473/LConn2 -- _CN_93147473_225000_CN_167908818_225000/LConn2
  _CN_271334706_225000_CN_93147473_225000/RConn3 -- T_93147473_400000;225000_/RConn3 -- _CN_93147473_225000_CN_131321800_225000/LConn3 -- _CN_93147473_225000_CN_131545712_225000/LConn3 -- L_93147473/LConn3 -- bus47/LConn1 -- _CN_93147473_225000_CN_167908818_225000/LConn3
  T_216888494_225000_/LConn1 -- _CN_216888494_225000_CN_207997682_225000/RConn1
  T_216888494_225000_/LConn2 -- _CN_216888494_225000_CN_207997682_225000/RConn2
  _CN_216888494_225000_CN_207997682_225000/RConn3 -- T_216888494_225000_/LConn3 -- bus48/LConn1
  T_166090341_225000;60000_/LConn1 -- _CN_143699506_225000_CN_166090341_225000/RConn1
  T_166090341_225000;60000_/LConn2 -- _CN_143699506_225000_CN_166090341_225000/RConn2
  _CN_143699506_225000_CN_166090341_225000/RConn3 -- T_166090341_225000;60000_/LConn3 -- bus49/LConn1
  _CN_131591106_225000_CN_143628748_225000/RConn1 -- T_131591106_225000_/LConn1 -- _CN_131591106_225000_CN_131588990_225000/RConn1
  _CN_131591106_225000_CN_143628748_225000/RConn2 -- T_131591106_225000_/LConn2 -- _CN_131591106_225000_CN_131588990_225000/RConn2
  _CN_131591106_225000_CN_143628748_225000/RConn3 -- T_131591106_225000_/LConn3 -- _CN_131591106_225000_CN_131588990_225000/RConn3 -- bus50/LConn1
  T_207823867__/LConn1 -- _CN_167406532_225000_CN_207823867_225000/RConn1
  T_207823867__/LConn2 -- _CN_167406532_225000_CN_207823867_225000/RConn2
  _CN_167406532_225000_CN_207823867_225000/RConn3 -- T_207823867__/LConn3 -- bus51/LConn1
  _CN_144011974_225000_CN_96831672_225000/RConn1 -- T_144011974_225000_/LConn1 -- _CN_144011974_225000_CN_197830862_225000/RConn1
  _CN_144011974_225000_CN_96831672_225000/RConn2 -- T_144011974_225000_/LConn2 -- _CN_144011974_225000_CN_197830862_225000/RConn2
  _CN_144011974_225000_CN_96831672_225000/RConn3 -- T_144011974_225000_/LConn3 -- _CN_144011974_225000_CN_197830862_225000/RConn3 -- bus52/LConn1
  _CN_131992905_225000_CN_207997682_225000/RConn1 -- T_131992905_225000_/LConn1 -- _CN_131992905_225000_CN_131995387_225000/RConn1 -- _CN_131992905_225000_CN_218859980_225000/LConn1
  _CN_131992905_225000_CN_207997682_225000/RConn2 -- T_131992905_225000_/LConn2 -- _CN_131992905_225000_CN_131995387_225000/RConn2 -- _CN_131992905_225000_CN_218859980_225000/LConn2
  _CN_131992905_225000_CN_207997682_225000/RConn3 -- T_131992905_225000_/LConn3 -- _CN_131992905_225000_CN_131995387_225000/RConn3 -- _CN_131992905_225000_CN_218859980_225000/LConn3 -- bus53/LConn1
  G_218859980_/RConn1 -- _CN_131992905_225000_CN_218859980_225000/RConn1
  G_218859980_/RConn2 -- _CN_131992905_225000_CN_218859980_225000/RConn2
  _CN_131992905_225000_CN_218859980_225000/RConn3 -- G_218859980_/RConn3 -- bus54/LConn1
  T_167908818_225000_/LConn1 -- _CN_93147473_225000_CN_167908818_225000/RConn1
  T_167908818_225000_/LConn2 -- _CN_93147473_225000_CN_167908818_225000/RConn2
  _CN_93147473_225000_CN_167908818_225000/RConn3 -- T_167908818_225000_/LConn3 -- bus55/LConn1
  _CN_93147473_225000_CN_131321800_225000/RConn1 -- G_131321800_/RConn1 -- _CN_93147473_400000_CN_131321800_225000/LConn1
  _CN_93147473_225000_CN_131321800_225000/RConn2 -- G_131321800_/RConn2 -- _CN_93147473_400000_CN_131321800_225000/LConn2
  _CN_93147473_225000_CN_131321800_225000/RConn3 -- G_131321800_/RConn3 -- _CN_93147473_400000_CN_131321800_225000/LConn3 -- bus56/LConn1
  T_131545712_225000;60000_/LConn1 -- _CN_93147473_225000_CN_131545712_225000/RConn1
  T_131545712_225000;60000_/LConn2 -- _CN_93147473_225000_CN_131545712_225000/RConn2
  _CN_93147473_225000_CN_131545712_225000/RConn3 -- T_131545712_225000;60000_/LConn3 -- bus57/LConn1
  T_131947753_225000_/LConn1 -- _CN_131902940_225000_CN_131947753_225000/RConn1
  T_131947753_225000_/LConn2 -- _CN_131902940_225000_CN_131947753_225000/RConn2
  _CN_131902940_225000_CN_131947753_225000/RConn3 -- T_131947753_225000_/LConn3 -- bus58/LConn1
  T_251222750_225000_/LConn1 -- _CN_95436126_225000_CN_251222750_225000/RConn1
  T_251222750_225000_/LConn2 -- _CN_95436126_225000_CN_251222750_225000/RConn2
  _CN_95436126_225000_CN_251222750_225000/RConn3 -- T_251222750_225000_/LConn3 -- bus59/LConn1
  G_150122664_/RConn1 -- _CN_143752299_225000_CN_150122664_225000/RConn1
  G_150122664_/RConn2 -- _CN_143752299_225000_CN_150122664_225000/RConn2
  _CN_143752299_225000_CN_150122664_225000/RConn3 -- G_150122664_/RConn3 -- bus60/LConn1
  T_97706499_225000_/LConn1 -- _CN_97706499_400000_CN_316738277_400000/LConn1
  T_97706499_225000_/LConn2 -- _CN_97706499_400000_CN_316738277_400000/LConn2
  _CN_97706499_400000_CN_316738277_400000/LConn3 -- T_97706499_225000_/LConn3 -- bus61/LConn1
  _CN_97706499_400000_CN_316738277_400000/RConn1 -- T_316738277__/LConn1 -- _CN_316738277_400000_CN_131946012_400000/LConn1
  _CN_97706499_400000_CN_316738277_400000/RConn2 -- T_316738277__/LConn2 -- _CN_316738277_400000_CN_131946012_400000/LConn2
  _CN_97706499_400000_CN_316738277_400000/RConn3 -- T_316738277__/LConn3 -- _CN_316738277_400000_CN_131946012_400000/LConn3 -- bus62/LConn1
  _CN_316738277_400000_CN_131946012_400000/RConn1 -- T_131946012_400000;225000_/LConn1 -- _CN_167920552_400000_CN_131946012_400000/LConn1
  _CN_316738277_400000_CN_131946012_400000/RConn2 -- T_131946012_400000;225000_/LConn2 -- _CN_167920552_400000_CN_131946012_400000/LConn2
  _CN_316738277_400000_CN_131946012_400000/RConn3 -- T_131946012_400000;225000_/LConn3 -- _CN_167920552_400000_CN_131946012_400000/LConn3 -- bus63/LConn1
  T_249897127_400000_/LConn1 -- _CN_249897127_400000_CN_93147473_400000/LConn1
  T_249897127_400000_/LConn2 -- _CN_249897127_400000_CN_93147473_400000/LConn2
  _CN_249897127_400000_CN_93147473_400000/LConn3 -- T_249897127_400000_/LConn3 -- bus64/LConn1
  _CN_249897127_400000_CN_93147473_400000/RConn1 -- T_93147473_400000;225000_/LConn1 -- _CN_167920552_400000_CN_93147473_400000/LConn1 -- _CN_93147473_400000_CN_131321800_225000/RConn1
  _CN_249897127_400000_CN_93147473_400000/RConn2 -- T_93147473_400000;225000_/LConn2 -- _CN_167920552_400000_CN_93147473_400000/LConn2 -- _CN_93147473_400000_CN_131321800_225000/RConn2
  _CN_249897127_400000_CN_93147473_400000/RConn3 -- T_93147473_400000;225000_/LConn3 -- _CN_167920552_400000_CN_93147473_400000/LConn3 -- _CN_93147473_400000_CN_131321800_225000/RConn3 -- bus65/LConn1
  _CN_167920552_400000_CN_93147473_400000/RConn1 -- T_167920552_400000;225000_/LConn1 -- _CN_167920552_400000_CN_131946012_400000/RConn1
  _CN_167920552_400000_CN_93147473_400000/RConn2 -- T_167920552_400000;225000_/LConn2 -- _CN_167920552_400000_CN_131946012_400000/RConn2
  _CN_167920552_400000_CN_93147473_400000/RConn3 -- T_167920552_400000;225000_/LConn3 -- _CN_167920552_400000_CN_131946012_400000/RConn3 -- bus66/LConn1
  T_200906153_225000_/RConn1 -- L_200906153/LConn1
  T_200906153_225000_/RConn2 -- L_200906153/LConn2
  L_200906153/LConn3 -- T_200906153_225000_/RConn3 -- bus67/LConn1
  T_250878457_225000_/RConn1 -- L_250878457/LConn1
  T_250878457_225000_/RConn2 -- L_250878457/LConn2
  L_250878457/LConn3 -- T_250878457_225000_/RConn3 -- bus68/LConn1
  T_285708473_225000_/RConn1 -- L_285708473/LConn1
  T_285708473_225000_/RConn2 -- L_285708473/LConn2
  L_285708473/LConn3 -- T_285708473_225000_/RConn3 -- bus69/LConn1
  T_218739270_225000_/RConn1 -- L_218739270/LConn1
  T_218739270_225000_/RConn2 -- L_218739270/LConn2
  L_218739270/LConn3 -- T_218739270_225000_/RConn3 -- bus70/LConn1
  T_271316486_225000_/RConn1 -- L_271316486/LConn1
  T_271316486_225000_/RConn2 -- L_271316486/LConn2
  L_271316486/LConn3 -- T_271316486_225000_/RConn3 -- bus71/LConn1
  T_215403934_225000_/RConn1 -- L_215403934/LConn1
  T_215403934_225000_/RConn2 -- L_215403934/LConn2
  L_215403934/LConn3 -- T_215403934_225000_/RConn3 -- bus72/LConn1
  T_320483882_225000_/RConn1 -- L_320483882/LConn1
  T_320483882_225000_/RConn2 -- L_320483882/LConn2
  L_320483882/LConn3 -- T_320483882_225000_/RConn3 -- bus73/LConn1
  T_200913450_225000_/RConn1 -- L_200913450/LConn1
  T_200913450_225000_/RConn2 -- L_200913450/LConn2
  L_200913450/LConn3 -- T_200913450_225000_/RConn3 -- bus74/LConn1
  T_182345278_225000_/RConn1 -- L_182345278/LConn1
  T_182345278_225000_/RConn2 -- L_182345278/LConn2
  L_182345278/LConn3 -- T_182345278_225000_/RConn3 -- bus75/LConn1
  T_94548360_225000_/RConn1 -- L_94548360/LConn1
  T_94548360_225000_/RConn2 -- L_94548360/LConn2
  L_94548360/LConn3 -- T_94548360_225000_/RConn3 -- bus76/LConn1
  T_208002693_225000_/RConn1 -- L_208002693/LConn1
  T_208002693_225000_/RConn2 -- L_208002693/LConn2
  L_208002693/LConn3 -- T_208002693_225000_/RConn3 -- bus77/LConn1
  T_108482559_225000_/RConn1 -- L_108482559/LConn1
  T_108482559_225000_/RConn2 -- L_108482559/LConn2
  L_108482559/LConn3 -- T_108482559_225000_/RConn3 -- bus78/LConn1
  T_131995387_225000_/RConn1 -- L_131995387/LConn1
  T_131995387_225000_/RConn2 -- L_131995387/LConn2
  L_131995387/LConn3 -- T_131995387_225000_/RConn3 -- bus79/LConn1
  T_131891079_225000;60000_/RConn1 -- L_131891079/LConn1
  T_131891079_225000;60000_/RConn2 -- L_131891079/LConn2
  L_131891079/LConn3 -- T_131891079_225000;60000_/RConn3 -- bus80/LConn1
  T_131892127_225000;60000_/RConn1 -- L_131892127/LConn1
  T_131892127_225000;60000_/RConn2 -- L_131892127/LConn2
  L_131892127/LConn3 -- T_131892127_225000;60000_/RConn3 -- bus81/LConn1
  T_207991977_225000_/RConn1 -- L_207991977/LConn1
  T_207991977_225000_/RConn2 -- L_207991977/LConn2
  L_207991977/LConn3 -- T_207991977_225000_/RConn3 -- bus82/LConn1
  T_131408509_225000_/RConn1 -- L_131408509/LConn1
  T_131408509_225000_/RConn2 -- L_131408509/LConn2
  L_131408509/LConn3 -- T_131408509_225000_/RConn3 -- bus83/LConn1
  T_131588990_225000;60000_/RConn1 -- L_131588990/LConn1
  T_131588990_225000;60000_/RConn2 -- L_131588990/LConn2
  L_131588990/LConn3 -- T_131588990_225000;60000_/RConn3 -- bus84/LConn1
  T_143628748_225000_/RConn1 -- L_143628748/LConn1
  T_143628748_225000_/RConn2 -- L_143628748/LConn2
  L_143628748/LConn3 -- T_143628748_225000_/RConn3 -- bus85/LConn1
  T_131902940_225000_/RConn1 -- L_131902940/LConn1
  T_131902940_225000_/RConn2 -- L_131902940/LConn2
  L_131902940/LConn3 -- T_131902940_225000_/RConn3 -- bus86/LConn1
  T_95436126_225000;60000_/RConn1 -- L_95436126/LConn1
  T_95436126_225000;60000_/RConn2 -- L_95436126/LConn2
  L_95436126/LConn3 -- T_95436126_225000;60000_/RConn3 -- bus87/LConn1
  T_163471767_225000_/RConn1 -- L_163471767/LConn1
  T_163471767_225000_/RConn2 -- L_163471767/LConn2
  L_163471767/LConn3 -- T_163471767_225000_/RConn3 -- bus88/LConn1
  T_143736898__/RConn1 -- L_143736898/LConn1
  T_143736898__/RConn2 -- L_143736898/LConn2
  L_143736898/LConn3 -- T_143736898__/RConn3 -- bus89/LConn1
  T_143752299_400000;225000_/RConn1 -- L_143752299/LConn1
  T_143752299_400000;225000_/RConn2 -- L_143752299/LConn2
  L_143752299/LConn3 -- T_143752299_400000;225000_/RConn3 -- bus90/LConn1
  T_167406532_225000_/RConn1 -- L_167406532/LConn1
  T_167406532_225000_/RConn2 -- L_167406532/LConn2
  L_167406532/LConn3 -- T_167406532_225000_/RConn3 -- bus91/LConn1
  T_143681023_225000;60000_/RConn1 -- L_143681023/LConn1
  T_143681023_225000;60000_/RConn2 -- L_143681023/LConn2
  L_143681023/LConn3 -- T_143681023_225000;60000_/RConn3 -- bus92/LConn1
  T_96831672_225000_/RConn1 -- L_96831672/LConn1
  T_96831672_225000_/RConn2 -- L_96831672/LConn2
  L_96831672/LConn3 -- T_96831672_225000_/RConn3 -- bus93/LConn1
  T_359251299__/RConn1 -- L_359251299/LConn1
  T_359251299__/RConn2 -- L_359251299/LConn2
  L_359251299/LConn3 -- T_359251299__/RConn3 -- bus94/LConn1
  T_208137370_225000_/RConn1 -- L_208137370/LConn1
  T_208137370_225000_/RConn2 -- L_208137370/LConn2
  L_208137370/LConn3 -- T_208137370_225000_/RConn3 -- bus95/LConn1
  T_144011573_225000;60000_/RConn1 -- L_144011573/LConn1
  T_144011573_225000;60000_/RConn2 -- L_144011573/LConn2
  L_144011573/LConn3 -- T_144011573_225000;60000_/RConn3 -- bus96/LConn1
  T_207995370__/RConn1 -- L_207995370/LConn1
  T_207995370__/RConn2 -- L_207995370/LConn2
  L_207995370/LConn3 -- T_207995370__/RConn3 -- bus97/LConn1
  T_207997682_225000;150000_/RConn1 -- L_207997682/LConn1
  T_207997682_225000;150000_/RConn2 -- L_207997682/LConn2
  L_207997682/LConn3 -- T_207997682_225000;150000_/RConn3 -- bus98/LConn1
  T_131899192__/RConn1 -- L_131899192/LConn1
  T_131899192__/RConn2 -- L_131899192/LConn2
  L_131899192/LConn3 -- T_131899192__/RConn3 -- bus99/LConn1
  T_131893727__/RConn1 -- L_131893727/LConn1
  T_131893727__/RConn2 -- L_131893727/LConn2
  L_131893727/LConn3 -- T_131893727__/RConn3 -- bus100/LConn1
  T_143685412_225000_/RConn1 -- L_143685412/LConn1
  T_143685412_225000_/RConn2 -- L_143685412/LConn2
  L_143685412/LConn3 -- T_143685412_225000_/RConn3 -- bus101/LConn1
  T_142520745__/RConn1 -- L_142520745/LConn1
  T_142520745__/RConn2 -- L_142520745/LConn2
  L_142520745/LConn3 -- T_142520745__/RConn3 -- bus102/LConn1
  T_200915133_225000_/RConn1 -- L_200915133/LConn1
  T_200915133_225000_/RConn2 -- L_200915133/LConn2
  L_200915133/LConn3 -- T_200915133_225000_/RConn3 -- bus103/LConn1
  T_197830862__/RConn1 -- L_197830862/LConn1
  T_197830862__/RConn2 -- L_197830862/LConn2
  L_197830862/LConn3 -- T_197830862__/RConn3 -- bus104/LConn1
  T_271334706__/RConn1 -- L_271334706/LConn1
  T_271334706__/RConn2 -- L_271334706/LConn2
  L_271334706/LConn3 -- T_271334706__/RConn3 -- bus105/LConn1
  T_143699506_225000_/RConn1 -- L_143699506/LConn1
  T_143699506_225000_/RConn2 -- L_143699506/LConn2
  L_143699506/LConn3 -- T_143699506_225000_/RConn3 -- bus106/LConn1
  T_216888494_225000_/RConn1 -- L_216888494/LConn1
  T_216888494_225000_/RConn2 -- L_216888494/LConn2
  L_216888494/LConn3 -- T_216888494_225000_/RConn3 -- bus107/LConn1
  T_166090341_225000;60000_/RConn1 -- L_166090341/LConn1
  T_166090341_225000;60000_/RConn2 -- L_166090341/LConn2
  L_166090341/LConn3 -- T_166090341_225000;60000_/RConn3 -- bus108/LConn1
  T_131591106_225000_/RConn1 -- L_131591106/LConn1
  T_131591106_225000_/RConn2 -- L_131591106/LConn2
  L_131591106/LConn3 -- T_131591106_225000_/RConn3 -- bus109/LConn1
  T_207823867__/RConn1 -- L_207823867/LConn1
  T_207823867__/RConn2 -- L_207823867/LConn2
  L_207823867/LConn3 -- T_207823867__/RConn3 -- bus110/LConn1
  T_144011974_225000_/RConn1 -- L_144011974/LConn1
  T_144011974_225000_/RConn2 -- L_144011974/LConn2
  L_144011974/LConn3 -- T_144011974_225000_/RConn3 -- bus111/LConn1
  T_131992905_225000_/RConn1 -- L_131992905/LConn1
  T_131992905_225000_/RConn2 -- L_131992905/LConn2
  L_131992905/LConn3 -- T_131992905_225000_/RConn3 -- bus112/LConn1
  T_167908818_225000_/RConn1 -- L_167908818/LConn1
  T_167908818_225000_/RConn2 -- L_167908818/LConn2
  L_167908818/LConn3 -- T_167908818_225000_/RConn3 -- bus113/LConn1
  T_131545712_225000;60000_/RConn1 -- L_131545712/LConn1
  T_131545712_225000;60000_/RConn2 -- L_131545712/LConn2
  L_131545712/LConn3 -- T_131545712_225000;60000_/RConn3 -- bus114/LConn1
  T_131947753_225000_/RConn1 -- L_131947753/LConn1
  T_131947753_225000_/RConn2 -- L_131947753/LConn2
  L_131947753/LConn3 -- T_131947753_225000_/RConn3 -- bus115/LConn1
  T_251222750_225000_/RConn1 -- L_251222750/LConn1
  T_251222750_225000_/RConn2 -- L_251222750/LConn2
  L_251222750/LConn3 -- T_251222750_225000_/RConn3 -- bus116/LConn1
  T_249897127_400000_/RConn1 -- L_249897127/LConn1
  T_249897127_400000_/RConn2 -- L_249897127/LConn2
  L_249897127/LConn3 -- T_249897127_400000_/RConn3 -- bus117/LConn1
